simulink model "FIR2"  (Simulink 6.6)
settings: Solver=ode45  StartTime=0.0  StopTime=2/f0  RelTol=1e-3
undefined symbols (not defined in the file or in its folder): dfilt, f0, Fe
libraries: dsparch4 x4
settings Model: Creator=chantal  LastModifiedBy=chantal

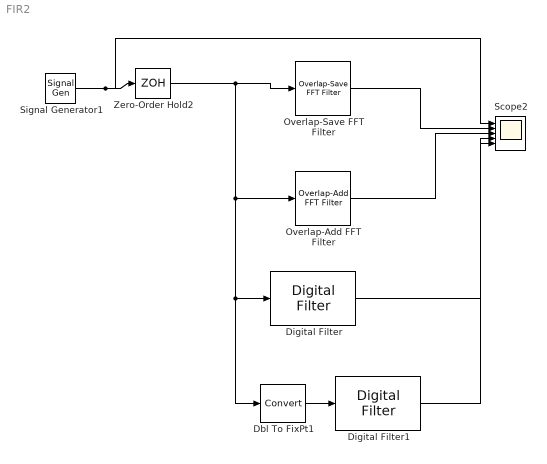
== system FIR2 ==
  Dbl To FixPt1 : DataTypeConversion  OutDataTypeMode=Specify via dialog  OutScaling=2^-13  RndMeth=Nearest  LockScale=on
  Digital Filter : dsparch4/Digital Filter  DialogController=dspdialog.DigitalFilter  DialogControllerArgs=DataTag0  TypePopup=FIR (all zeros)  IIRFiltStruct=Direct form II transposed  AllPoleFiltStruct=Direct form  FIRFiltStruct=Direct form  CoeffSource=Specify via dialog  NumCoeffs=1/32*ones(1,32)  DenCoeffs=[1 0.1]  BiQuadCoeffs=[1 0.3 0.4 1 0.1 0.2]  LatticeCoeffs=[0.2 0.4]  denIgnore=on  FiltPerSampPopup=One filter per frame  IC=0  ICnum=0  ICden=0  roundingMode=Floor  overflowMode=off  ScaleValues=1  scaleValueFracLength=14  stageInFracLength=15  stageOutFracLength=15  FilterSource=Specify via dialog  dfiltObjectName=dfilt.dffir([1 2 1])
  Digital Filter1 : dsparch4/Digital Filter  DialogController=dspdialog.DigitalFilter  DialogControllerArgs=DataTag1  TypePopup=FIR (all zeros)  IIRFiltStruct=Direct form II transposed  AllPoleFiltStruct=Direct form  FIRFiltStruct=Direct form  CoeffSource=Specify via dialog  NumCoeffs=1/32*ones(1,32)  DenCoeffs=[1 0.1]  BiQuadCoeffs=[1 0.3 0.4 1 0.1 0.2]  LatticeCoeffs=[0.2 0.4]  denIgnore=on  FiltPerSampPopup=One filter per frame  IC=0  ICnum=0  ICden=0  firstCoeffMode=Binary point scaling  firstCoeffWordLength=16  firstCoeffFracLength=15  prodOutputMode=Binary point scaling  prodOutputWordLength=32  prodOutputFracLength=28  roundingMode=Floor  overflowMode=on  ScaleValues=1  scaleValueFracLength=14  stageInFracLength=15  stageOutFracLength=15  FilterSource=Specify via dialog  dfiltObjectName=dfilt.dffir([1 2 1])
      settings: LockScale=on
  Overlap-Add FFT Filter : dsparch4/Overlap-Add FFT Filter  SystemSampleTime=-1  Nfft=128  h=1/32*ones(1,32)  output_complexity=Real
  Overlap-Save FFT Filter : dsparch4/Overlap-Save FFT Filter  SystemSampleTime=-1  nfft_in=128  h=1/32*ones(1,32)  output_complexity=Real
  Scope2 : Scope  NumInputPorts=5
      settings: YMin=-5~-5~-5~-5~-5  YMax=5~5~5~5~5
  Signal Generator1 : SignalGenerator  Amplitude=32  Frequency=f0
  Zero-Order Hold2 : ZeroOrderHold  SampleTime=1/Fe
  wires:
  Signal Generator1/1 -> Zero-Order Hold2/1, Scope2/1
  Zero-Order Hold2/1 -> Overlap-Save FFT Filter/1, Overlap-Add FFT Filter/1, Digital Filter/1, Dbl To FixPt1/1
  Overlap-Save FFT Filter/1 -> Scope2/2
  Overlap-Add FFT Filter/1 -> Scope2/3
  Digital Filter/1 -> Scope2/4
  Digital Filter1/1 -> Scope2/5
  Dbl To FixPt1/1 -> Digital Filter1/1
